simulink model "drone_controller"  (R2020b)
settings: Solver=VariableStepAuto  StartTime=0.0  StopTime=15.0  RelTol=1e-3
values from neighbouring files (symbols this model uses):
  b = 0.5    [run_sim.m]
  d = 0.5    [run_sim.m]
  I = [Ix, 0, 0 ... (first row only)    [run_sim.m]
  J_TP = 0.5    [run_sim.m]
  l = 0.2    [run_sim.m]
  m = 5    [run_sim.m]
  psi_t = 0.7    [run_sim.m]
  Q_a = [100000,0,0,0,0,0 ... (first row only)    [run_sim.m]
  Q_p = [1,0,0,0 ... (first row only)    [run_sim.m]
  Q_z = [1000,0 ... (first row only)    [run_sim.m]
  R_a = 10    [run_sim.m]
  R_p = 20    [run_sim.m]
  R_z = 1    [run_sim.m]
  x_t = 1    [run_sim.m]
  y_t = 2    [run_sim.m]
  z_t = 5    [run_sim.m]
settings Model: OrderedModelArguments=off  Creator=Peter Guglielmino  LastModifiedBy=Peter Guglielmino

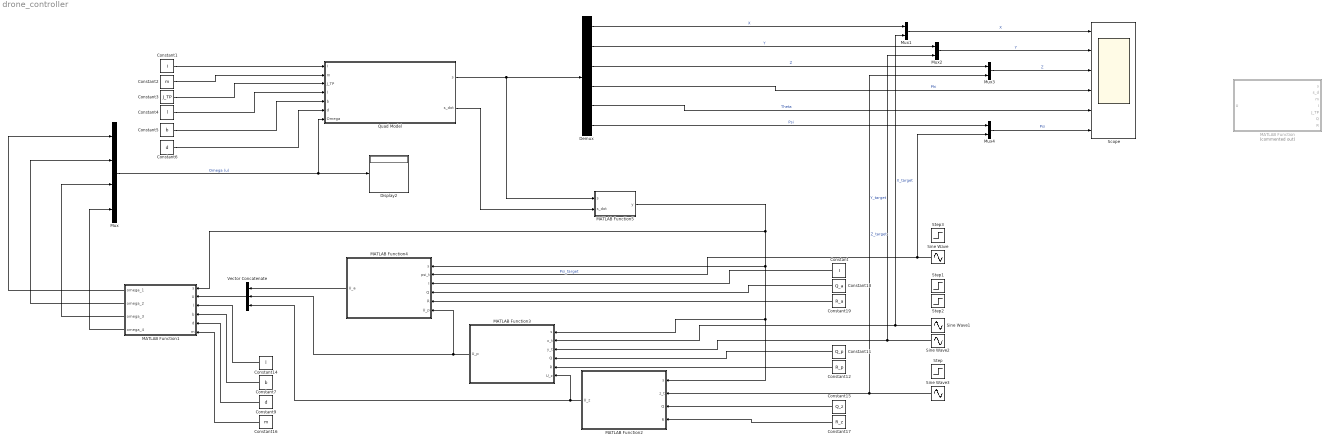
== system drone_controller ==
  Constant : Constant  Value=I
  Constant1 : Constant  Value=I
  Constant11 : Constant  Value=Q_p
  Constant12 : Constant  Value=R_p
  Constant14 : Constant  Value=l
  Constant15 : Constant  Value=Q_z
  Constant16 : Constant  Value=m
  Constant17 : Constant  Value=R_z
  Constant18 : Constant  Value=Q_a
  Constant19 : Constant  Value=R_a
  Constant2 : Constant  Value=m
  Constant3 : Constant  Value=J_TP
  Constant4 : Constant  Value=l
  Constant5 : Constant  Value=b
  Constant6 : Constant  Value=d
  Constant7 : Constant  Value=b
  Constant9 : Constant  Value=d
  Demux : Demux  Outputs=6
  Display2 : Display
  MATLAB Function : MATLAB Function  Commented=on  TreatAsAtomicUnit=on
  MATLAB Function1 : MATLAB Function  TreatAsAtomicUnit=on
  MATLAB Function2 : MATLAB Function  TreatAsAtomicUnit=on
  MATLAB Function3 : MATLAB Function  TreatAsAtomicUnit=on
  MATLAB Function4 : MATLAB Function  TreatAsAtomicUnit=on
  MATLAB Function5 : MATLAB Function  TreatAsAtomicUnit=on
  Mux : Mux
  Mux{1..4} (4 alike) : Mux  Inputs=2
  Quad Model : Subsystem
  Scope : Scope  NumInputPorts=6
  Sine Wave : Sin  Amplitude=psi_t  Frequency=0.5  SampleTime=0
  Sine Wave1 : Sin  Amplitude=x_t  Frequency=0.5  SampleTime=0
  Sine Wave2 : Sin  Amplitude=y_t  Frequency=0.5  SampleTime=0
  Sine Wave3 : Sin  Amplitude=z_t  Frequency=0.5  SampleTime=0
  Step : Step  Time=0  After=z_t  SampleTime=0
  Step1 : Step  Time=0  After=x_t  SampleTime=0
  Step2 : Step  Time=0  After=y_t  SampleTime=0
  Step3 : Step  Time=0  After=psi_t  SampleTime=0
  Vector Concatenate : Concatenate  NumInputs=3
  wires:
  Constant1/1 -> Quad Model/1(I)
  Constant2/1 -> Quad Model/2(m)
  Constant3/1 -> Quad Model/3(J_TP)
  Constant4/1 -> Quad Model/4(l)
  Constant5/1 -> Quad Model/5(b)
  Constant6/1 -> Quad Model/6(d)
  Quad Model/1(s) -> MATLAB Function5/1(s), Demux/1
  Demux/1 -> Mux1/1  "X"
  Demux/2 -> Mux2/1  "Y"
  Demux/3 -> Mux3/1  "Z"
  Demux/4 -> Scope/4  "Phi"
  Demux/5 -> Scope/5  "Theta"
  Demux/6 -> Mux4/1  "Psi"
  MATLAB Function1/1(omega_1) -> Mux/1
  MATLAB Function1/2(omega_2) -> Mux/2
  MATLAB Function1/3(omega_3) -> Mux/3
  MATLAB Function1/4(omega_4) -> Mux/4
  Constant7/1 -> MATLAB Function1/4(b)
  Constant9/1 -> MATLAB Function1/5(d)
  Constant14/1 -> MATLAB Function1/3(l)
  Quad Model/2(s_dot) -> MATLAB Function5/2(s_dot)
  Mux/1 -> Quad Model/7(Omega), Display2/1  "Omega (u)"
  Constant/1 -> MATLAB Function4/3(I)
  Sine Wave/1 -> MATLAB Function4/2(psi_t), Mux4/2  "Psi_target"
  MATLAB Function5/1(y) -> MATLAB Function1/1(s), MATLAB Function4/1(s), MATLAB Function2/1(s), MATLAB Function3/1(s)
  Constant16/1 -> MATLAB Function1/6(m)
  MATLAB Function3/1(U_p) -> Vector Concatenate/2, MATLAB Function4/6(U_p)
  Vector Concatenate/1 -> MATLAB Function1/2(U)
  MATLAB Function4/1(U_a) -> Vector Concatenate/1
  MATLAB Function2/1(U_z) -> Vector Concatenate/3, MATLAB Function3/6(U_z)
  Sine Wave1/1 -> MATLAB Function3/2(x_t), Mux1/2  "X_target"
  Constant11/1 -> MATLAB Function3/4(Q)
  Constant12/1 -> MATLAB Function3/5(R)
  Constant17/1 -> MATLAB Function2/4(R)
  Constant15/1 -> MATLAB Function2/3(Q)
  Constant18/1 -> MATLAB Function4/4(Q)
  Constant19/1 -> MATLAB Function4/5(R)
  Sine Wave3/1 -> Mux3/2, MATLAB Function2/2(z_t)  "Z_target"
  Sine Wave2/1 -> Mux2/2, MATLAB Function3/3(y_t)  "Y_target"
  Mux1/1 -> Scope/1  "X"
  Mux2/1 -> Scope/2  "Y"
  Mux3/1 -> Scope/3  "Z"
  Mux4/1 -> Scope/6  "Psi"

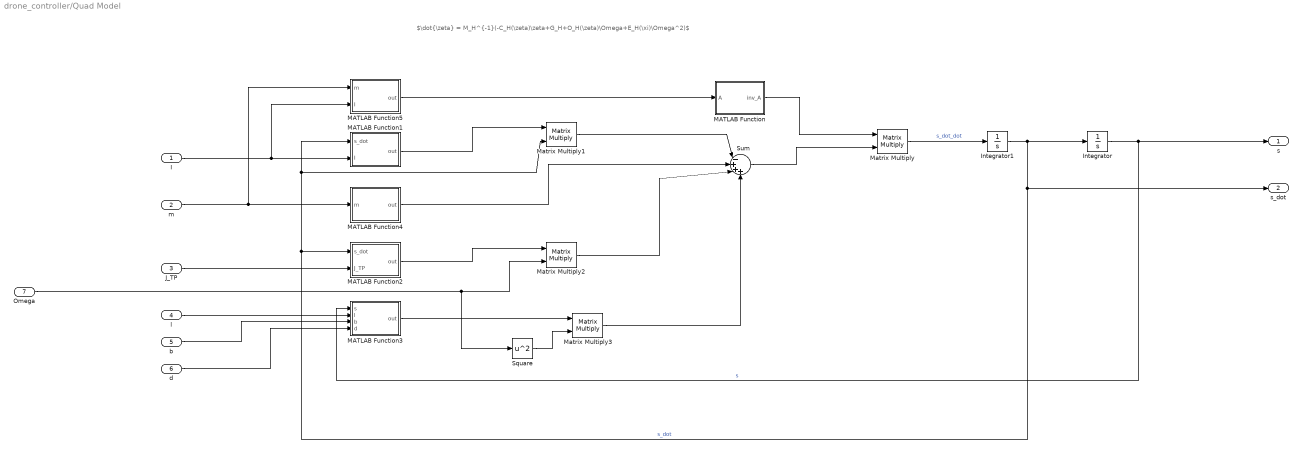
== system drone_controller/Quad Model ==
  note: $\dot{\zeta} = M_H^{-1}(-C_H(\zeta)\zeta+G_H+O_H(\zeta)\Omega+E_H(\xi)\Omega^2)$
  I : Inport
  m : Inport  Port=2
  J_TP : Inport  Port=3
  l : Inport  Port=4
  b : Inport  Port=5
  d : Inport  Port=6
  Omega : Inport  Port=7
  Integrator : Integrator
  Integrator1 : Integrator
  MATLAB Function : MATLAB Function  TreatAsAtomicUnit=on
  MATLAB Function1 : MATLAB Function  TreatAsAtomicUnit=on
  MATLAB Function2 : MATLAB Function  TreatAsAtomicUnit=on
  MATLAB Function3 : MATLAB Function  TreatAsAtomicUnit=on
  MATLAB Function4 : MATLAB Function  TreatAsAtomicUnit=on
  MATLAB Function5 : MATLAB Function  TreatAsAtomicUnit=on
  Matrix Multiply{,1..3} (4 alike) : Product  Multiplication=Matrix(*)
  Square : Math  Operator=square  SaturateOnIntegerOverflow=on
  Sum : Sum  Inputs=|-+++
  s : Outport
  s_dot : Outport  Port=2
  wires:
  Square/1 -> Matrix Multiply3/2
  MATLAB Function/1(inv_A) -> Matrix Multiply/1
  b/1 -> MATLAB Function3/3(b)
  I/1 -> MATLAB Function5/2(I), MATLAB Function1/2(I)
  MATLAB Function5/1(out) -> MATLAB Function/1(A)
  Matrix Multiply1/1 -> Sum/1
  Integrator/1 -> s/1, MATLAB Function3/1(s)  "s"
  J_TP/1 -> MATLAB Function2/2(J_TP)
  m/1 -> MATLAB Function5/1(m), MATLAB Function4/1(m)
  Integrator1/1 -> s_dot/1, MATLAB Function2/1(s_dot), Matrix Multiply1/2, MATLAB Function1/1(s_dot), Integrator/1  "s_dot"
  Sum/1 -> Matrix Multiply/2
  MATLAB Function3/1(out) -> Matrix Multiply3/1
  Matrix Multiply/1 -> Integrator1/1  "s_dot_dot"
  MATLAB Function4/1(out) -> Sum/2
  Omega/1 -> Square/1, Matrix Multiply2/2
  MATLAB Function2/1(out) -> Matrix Multiply2/1
  Matrix Multiply2/1 -> Sum/3
  Matrix Multiply3/1 -> Sum/4
  MATLAB Function1/1(out) -> Matrix Multiply1/1
  l/1 -> MATLAB Function3/2(l)
  d/1 -> MATLAB Function3/4(d)

== matlab function drone_controller/MATLAB Function3 ==
  data: s input; U_p output; x_t input; y_t input; Q input; R input; U_z input
function U_p = position_control(s, x_t, y_t, Q, R, U_z)

% s = [x, dx, y, dy, z, dz, phi, p, theta, q, psi, r]

coder.extrinsic('lqr');

x = s(1:4);
x_d = [x_t;0;y_t;0];

g = 9.8;
a = U_z + g;

A = [0,1,0,0;
     0,0,0,0;
     0,0,0,1;
     0,0,0,0];
 
B = [0,0;
     a,0;
     0,0;
     0,a];
  
C = [1,0,0,0;
     0,0,1,0];

r = C*x_d;

K = zeros(2,4);

[K,S,e] = lqr(A, B, Q, R);

k_r = -inv(C/(A-B*K)*B);

U_p = -K*x + k_r*r;

== matlab function drone_controller/MATLAB Function4 ==
  data: s input; psi_t input; U_a output; I input; Q input; R input; U_p input
function U_a = attitude_control(s, psi_t, I, Q, R, U_p)

% s = [x, dx, y, dy, z, dz, !phi, p, theta, q, psi, r!]
% U_p = [U_x, U_y]
% U_x = (cos(phi)*sin(theta)*cos(psi) + sin(phi)*sin(psi))/(cos(phi)*cos(theta))
% U_y = (cos(phi)*sin(theta)*sin(psi) - sin(phi)*cos(psi))/(cos(phi)*cos(theta))
% theta = atan2(U_y + U_x*tan(psi),sin(psi)-cos(psi)^2)
% phi = atan2(U_x*cos(theta)-sin(theta)*cos(psi),sin(psi))

coder.extrinsic('lqr');

Ix = I(1);
Iy = I(5);
Iz = I(9);

x = s(7:12);

U_x = U_p(1);
U_y = U_p(2);

psi = x(5);
K = U_x^2 + U_y^2;

if (U_x^2 + U_y^2) == 0
    phi = 0;
else
    phi = asin(sqrt(K/((1+K)*(U_x^2+U_y^2))) * (U_x*sin(psi) - U_y*cos(psi)));
end

s = sign(U_y*sin(psi) + U_x*cos(psi));
if abs(1/(cos(phi)*sqrt(1+K))) > 1
    theta = s*acos(sign(1/(cos(phi)*sqrt(1+K))));
else
    theta = s*acos(1/(cos(phi)*sqrt(1+K)));
end

% theta = s*acos(1/(cos(phi)*sqrt(1+K)));


x_d = [phi; 0; theta; 0; psi_t; 0];

A = [0,1,0,0,0,0;
     0,0,0,0,0,0;
     0,0,0,1,0,0;
     0,0,0,0,0,0;
     0,0,0,0,0,1;
     0,0,0,0,0,0];
 
B = [0,0,0;
     (1/Ix),0,0;
     0,0,0;
     0,(1/Iy),0;
     0,0,0;
     0,0,(1/Iz)];
 
C = [1,0,0,0,0,0;
     0,0,1,0,0,0;
     0,0,0,0,1,0];
 
r = C*x_d;

K = zeros(3,6);

[K,S,e] = lqr(A, B, Q, R);

k_r = -inv(C/(A-B*K)*B);

U_a = -K*x + k_r*r;

== matlab function drone_controller/MATLAB Function5 ==
  data: s input; y output; s_dot input
function y = mixer(s, s_dot)

x = [s(1);s_dot(1);s(2);s_dot(2);s(3);s_dot(3);s(4);s_dot(4);s(5);s_dot(5);s(6);s_dot(6)];

y = x;

== matlab function drone_controller/Quad Model/MATLAB Function1 ==
  data: s_dot input; out output; I input
function out = C_H(s_dot, I)
% s_dot is the current change in state of the quadcopter
% I is the inertia matrix

skew = I*s_dot(4:6);

out = [zeros(3,3), zeros(3,3);
       zeros(1,3), 0, -skew(3), skew(2);
       zeros(1,3), skew(3), 0, -skew(1);
       zeros(1,3), -skew(2), skew(1), 0];

== matlab function drone_controller/Quad Model/MATLAB Function ==
  data: A input; inv_A output
function inv_A = m_inverse(A)
inv_A = inv(A);

== matlab function drone_controller/Quad Model/MATLAB Function2 ==
  data: s_dot input; out output; J_TP input
function out = O_H(s_dot, J_TP)
% s_dot is the current change in state of the quadcopter
% J_TP is the motor moment

p = s_dot(4);
q = s_dot(5);

O = [zeros(3,4);
     q, -q, q, -q;
     -p, p, -p, p;
     0, 0, 0, 0];

out = J_TP*O;

== matlab function drone_controller/Quad Model/MATLAB Function3 ==
  data: s input; out output; l input; b input; d input
function out = E_H(s, l, b, d)
% s is the current state of the quadcopter
% l is the length of the propellor blades
% b is the thrust constant
% d is the drag constant

phi = s(4);
theta = s(5);
psi = s(6);

R = [cos(psi)*cos(theta), -sin(psi)*cos(phi) + cos(psi)*sin(theta)*sin(phi), sin(psi)*sin(phi) + cos(psi)*sin(theta)*cos(phi);
     sin(psi)*cos(theta), cos(psi)*cos(phi) + sin(psi)*sin(theta)*sin(phi), -cos(psi)*sin(phi) + sin(psi)*sin(theta)*cos(phi);
     -sin(theta), cos(theta)*sin(phi), cos(theta)*cos(phi)];

E_B = [zeros(2,4);
       b, b, b, b;
       0, -b*l, 0, b*l;
       -b*l, 0, b*l, 0;
       -d, d, -d, d];
       
T = [R, zeros(3,3);
    zeros(3,3), eye(3)];


out = T*E_B;

== matlab function drone_controller/Quad Model/MATLAB Function4 ==
  data: m input; out output
function out = G_H(m)
% m is the mass of the drone

g = 9.8;

out = [0;
       0;
       -m*g;
       0;
       0;
       0];

== matlab function drone_controller/Quad Model/MATLAB Function5 ==
  data: m input; out output; I input
function out = M_H(m, I)
% m is the mass of the quadcopter
% I is the inertia matrix

out = [m, 0, 0, 0, 0, 0;
       0, m, 0, 0, 0, 0;
       0, 0, m, 0, 0, 0;
       zeros(3,3), I];

== matlab function drone_controller/MATLAB Function ==
  data: s input; U output; s_d input; m input; I input; J_TP input; Q input; R input
function U = LQR(s, s_d, m, I, J_TP, Q, R)
% s_d = [x_d, 0, y_d, 0, z_d, 0, 0, 0, 0, 0, psi_d, 0]

coder.extrinsic('lqr');

Ix = I(1);
Iy = I(5);
Iz = I(9);

x = s(1);
y = s(3);
z = s(5);
psi = s(11);

theta = 0;
phi = 0;
q = 0;
r = 0;
p = 0;

g = 9.8;

U1 = m*g;
U2 = 0;
U3 = 0;
U4 = 0;
Omega = 0;

U_ss = [U1; U2; U3; U4; Omega];

A = [ 0, 1, 0, 0, 0, 0,                                                          0,       0,                                   0,        0,                                                         0, 0;
    0, 0, 0, 0, 0, 0,  (U1*(cos(phi)*sin(psi) - cos(psi)*sin(phi)*sin(theta)))/5,       0, (U1*cos(phi)*cos(psi)*cos(theta))/5,        0, (U1*(cos(psi)*sin(phi) - cos(phi)*sin(psi)*sin(theta)))/5, 0;
    0, 0, 0, 1, 0, 0,                                                          0,       0,                                   0,        0,                                                         0, 0;
    0, 0, 0, 0, 0, 0, -(U1*(cos(phi)*cos(psi) + sin(phi)*sin(psi)*sin(theta)))/5,       0, (U1*cos(phi)*cos(theta)*sin(psi))/5,        0, (U1*(sin(phi)*sin(psi) + cos(phi)*cos(psi)*sin(theta)))/5, 0;
    0, 0, 0, 0, 0, 1,                                                          0,       0,                                   0,        0,                                                         0, 0;
    0, 0, 0, 0, 0, 0,                                -(U1*cos(theta)*sin(phi))/5,       0,         -(U1*cos(phi)*sin(theta))/5,        0,                                                         0, 0;
    0, 0, 0, 0, 0, 0,                                                          0,       1,                                   0,        0,                                                         0, 0;
    0, 0, 0, 0, 0, 0,                                                          0,       0,                                   0, -5*Omega,                                                         0, 0;
    0, 0, 0, 0, 0, 0,                                                          0,       0,                                   0,        1,                                                         0, 0;
    0, 0, 0, 0, 0, 0,                                                          0, 5*Omega,                                   0,        0,                                                         0, 0;
    0, 0, 0, 0, 0, 0,                                                          0,       0,                                   0,        0,                                                         0, 1;
    0, 0, 0, 0, 0, 0,                                                          0,       0,                                   0,        0,                                                         0, 0];

% a1 = ((Iy-Iz)/Ix)*r - J_TP/Ix*Omega;
% a2 = ((Iz-Ix)/Iy)*r + J_TP/Iy*Omega;
% a3 = ((Ix-Iy)/Iz)*q;
% 
% A = [0,1,0,0,0,0,0,0,0,0,0,0;
%      0,0,0,0,0,0,0,0,0,0,0,0;
%      0,0,0,1,0,0,0,0,0,0,0,0;
%      0,0,0,0,0,0,0,0,0,0,0,0;
%      0,0,0,0,0,1,0,0,0,0,0,0;
%      0,0,0,0,0,0,0,0,0,0,0,0;
%      0,0,0,0,0,0,0,1,0,0,0,0;
%      0,0,0,0,0,0,0,0,0,a1,0,0;
%      0,0,0,0,0,0,0,0,0,1,0,0;
%      0,0,0,0,0,0,0,a2,0,0,0,0;
%      0,0,0,0,0,0,0,0,0,0,0,1;
%      0,0,0,0,0,0,0,a3,0,0,0,0];
 
B = [0,  0,  0,  0,    0;
    (sin(phi)*sin(psi))/5 + (cos(phi)*cos(psi)*sin(theta))/5,  0,  0,  0,    0;
    0,  0,  0,  0,    0;
    (cos(phi)*sin(psi)*sin(theta))/5 - (cos(psi)*sin(phi))/5,  0,  0,  0,    0;
    0,  0,  0,  0,    0;
    (cos(phi)*cos(theta))/5,  0,  0,  0,    0;
    0,  0,  0,  0,    0;
    0, 10,  0,  0, -5*q;
    0,  0,  0,  0,    0;
    0,  0, 10,  0,  5*p;
    0,  0,  0,  0,    0;
    0,  0,  0, 10,    0];

% b1 = (sin(psi)*sin(phi) + cos(psi)*sin(theta)*cos(phi))/m;
% b2 = (-cos(psi)*sin(phi) + sin(psi)*sin(theta)*cos(phi))/m;
% b3 = (cos(theta)*cos(phi))/m;
% b4 = 1/Ix;
% b5 = 1/Iy;
% b6 = 1/Iz;
% 
% B = [0,0,0,0,0;
%      b1,0,0,0,0;
%      0,0,0,0,0;
%      b2,0,0,0,0;
%      0,0,0,0,0;
%      b3,0,0,0,0;
%      0,0,0,0,0;
%      0,b4,0,0,0;
%      0,0,0,0,0;
%      0,0,b5,0,0;
%      0,0,0,0,0;
%      0,0,0,0,b6];

K = zeros(5,12);

[K,S,e] = lqr(A, B, Q, R);

ds = s_d - s;

U = U_ss - K*ds;

== matlab function drone_controller/MATLAB Function1 ==
  data: s input; U input size=6; l input; omega_1 output; omega_2 output; omega_3 output; omega_4 output; b input; d input; m input
function [omega_1, omega_2, omega_3, omega_4] = U_to_Omega(s, U, l, b, d, m)

% s = [x, dx, y, dy, z, dz, phi, p, theta, q, psi, r]
% U = [U2, U3, U4, Ux, Uy, Uz]
% U1 = b*(omega_1^2 + omega_2^2 + omega_3^2 + omega_4^2)
% U2 = lb*(-omega_2^2 + omega_4^2)
% U3 = lb*(-omega_1^2 + omega_3^2)
% U4 = d*(-omega_1^2 + omega_2^2 - omega_3^2 + omega_4^2)
% Ux = cos(phi)sin(theta)cos(psi) + sin(phi)cos(psi)
% Uy = cos(phi)sin(theta)sin(psi) - sin(phi)cos(psi)
% Uz = g + (cos(phi)cos(theta))*1/m*U1


phi = s(7);
theta = s(9);

g = 9.8;

U1 = m*(U(6) + g)/(cos(phi)*cos(theta));

U_n = U(1:3);
U_n = [U1; U_n];

A = [b, b, b, b;
     0, -l*b, 0, l*b;
     -l*b, 0, l*b, 0;
     -d, d, -d, d];
O_sqr = A\U_n;

if (O_sqr(1) > 0)
    omega_1 = sqrt(O_sqr(1));
else
    omega_1 = 0;
end

if (O_sqr(2) > 0)
    omega_2 = sqrt(O_sqr(2));
else
    omega_2 = 0;
end

if (O_sqr(3) > 0)
    omega_3 = sqrt(O_sqr(3));
else
    omega_3 = 0;
end

if (O_sqr(4) > 0)
    omega_4 = sqrt(O_sqr(4));
else
    omega_4 = 0;
end

== matlab function drone_controller/MATLAB Function2 ==
  data: s input; z_t input; Q input; R input; U_z output
function U_z = altitude_control(s, z_t, Q, R)

% s = [x, dx, y, dy, z, dz, phi, p, theta, q, psi, r]

coder.extrinsic('lqr');

x = s(5:6);
x_d = [z_t; 0];

A = [0,1;
     0,0];
 
B = [0;1];

C = [1,0];

r = C*x_d;

K = zeros(1,2);

[K,S,e] = lqr(A, B, Q, R);

k_r = -inv(C/(A-B*K)*B);

U_z = -K*x + k_r*r;
